simulink model "simulacao"  (R2020a)
settings: Solver=VariableStepAuto  StartTime=0.0  StopTime=10.0  RelTol=1e-3
undefined symbols (not defined in the file): A, B, K
settings Model: Creator=valac  LastModifiedBy=valac

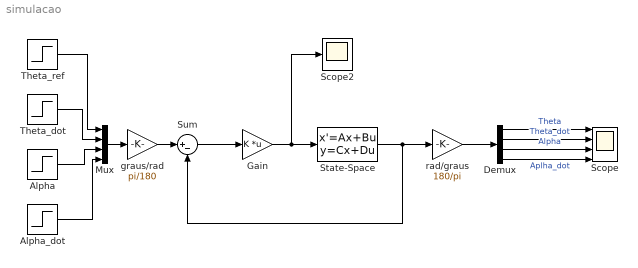
== system simulacao ==
  Alpha : Step  Time=0.5  After=0  SampleTime=0
  Alpha_dot : Step  After=0  SampleTime=0
  Demux : Demux
  Gain : Gain  Gain=K  Multiplication=Matrix(K*u)
  Mux : Mux
  Scope : Scope  NumInputPorts=4
  Scope2 : Scope
  State-Space : StateSpace  A=A  B=B  C=eye(4)  D=zeros(4,1)  InitialCondition=0
  Sum : Sum  Inputs=|+-
  Theta_dot : Step  After=0  SampleTime=0
  Theta_ref : Step  After=60  SampleTime=0
  graus/rad : Gain  Gain=pi/180
  rad/graus : Gain  Gain=180/pi
  wires:
  Sum/1 -> Gain/1
  Demux/1 -> Scope/1  "Theta"
  Demux/2 -> Scope/2  "Theta_dot"
  State-Space/1 -> rad/graus/1, Sum/2
  Demux/3 -> Scope/3  "Alpha"
  Demux/4 -> Scope/4  "Aplha_dot"
  Gain/1 -> State-Space/1, Scope2/1
  Theta_dot/1 -> Mux/2
  Alpha_dot/1 -> Mux/4
  Alpha/1 -> Mux/3
  Theta_ref/1 -> Mux/1
  Mux/1 -> graus/rad/1
  rad/graus/1 -> Demux/1
  graus/rad/1 -> Sum/1
